simulink model "try01"  (R2020b)
settings: Solver=VariableStepAuto  StartTime=0.0  StopTime=5  FixedStep=1e-4  RelTol=10e-1  AbsTol=1e-1
settings Model: SimulationMode=accelerator  Creator=engwe  LastModifiedBy=engwe
settings OptimizationCC: DefaultParameterBehavior=Inlined  UseDivisionForNetSlopeComputation=on  GainParamInheritBuiltInType=on  UseFloatMulNetSlope=on  InlineInvariantSignals=on  ZeroExternalMemoryAtStartup=off  ZeroInternalMemoryAtStartup=off  EfficientFloat2IntCast=on  LifeSpan=1
settings HardwareCC: ProdLongLongMode=on
settings SFSimCC: MATLABDynamicMemAlloc=off
settings RTWCC: GenerateReport=on  BuildConfiguration=Faster Runs  LaunchReport=on  TargetLang=C++
settings CodeAppCC: ForceParamTrailComments=on
settings GRTTargetCC: TargetLangStandard=C++03 (ISO)  CombineSignalStateStructs=on  MatFileLogging=off  CodeInterfacePackaging=C++ class  SupportVariableSizeSignals=on

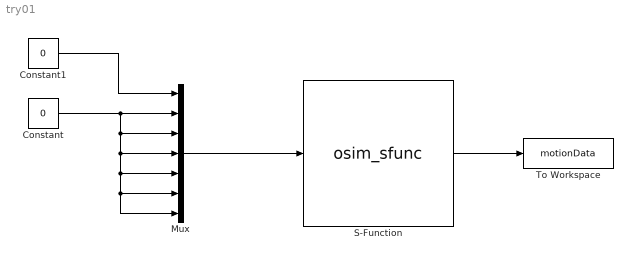
== system try01 ==
  Constant : Constant  Value=0
  Constant1 : Constant  Value=0
  Mux : Mux  Inputs=7
  S-Function : S-Function  FunctionName=osim_sfunc  SFunctionDeploymentMode=off  EnableBusSupport=off
      mask Display: image('mask.png'); % Use "Edit Image" on toolstrip to change.
  To Workspace : ToWorkspace  VariableName=motionData  SaveFormat=Timeseries  SampleTime=-1
  wires:
  S-Function/1 -> To Workspace/1
  Mux/1 -> S-Function/1
  Constant/1 -> Mux/7, Mux/6, Mux/5, Mux/4, Mux/3, Mux/2
  Constant1/1 -> Mux/1
